simulink model "phi4_m2_vr001_k5_3"  (R2021a)
settings: Solver=FixedStepAuto  StartTime=0.0  StopTime=24.0  FixedStep=1.0  RelTol=1e-3
libraries: deeplib x1
settings Model: Creator=ldy  LastModifiedBy=ldy
settings DataIOCC: SaveFormat=Array  SignalLogging=off  DSMLogging=off
settings DebuggingCC: UnconnectedInputMsg=none  UnconnectedOutputMsg=none  UnconnectedLineMsg=none
settings ModelReferenceCC: EnableRefExpFcnMdlSchedulingChecks=off
settings RTWCC: Description=Generic Real-Time Target  GPUComputeCapability=5.0  DLArmComputeVersion=20.02.1

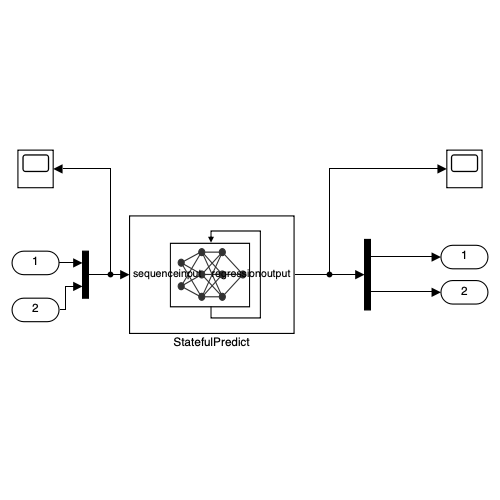
[thumbnail: Simulink's stored preview of the top-level diagram]
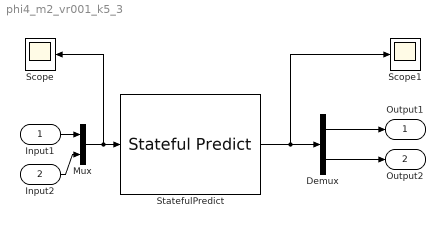
== system phi4_m2_vr001_k5_3 ==
  Input1 : Inport
  Input2 : Inport  Port=2
  Demux : Demux  Outputs=2
  Mux : Mux  Inputs=2
  Scope : Scope
  Scope1 : Scope
  StatefulPredict : deeplib/Stateful Predict  Network=Network from MAT-file  NetworkFunction=untitled  NetworkFilePath=SB4-Synthetic_Benchmark_4/phi4_m2_vr001_k5_3.mat  InputDataFormats={'',''}  SampleTime=1  ForceInterpretedSim=off  EnableDLNetwork=on  LastKnownNetworkFilePath=''  LastKnownNetworkTimeStamp=''
  Output1 : Outport
  Output2 : Outport  Port=2
  wires:
  Input1/1 -> Mux/1
  Input2/1 -> Mux/2
  Mux/1 -> Scope/1, StatefulPredict/1
  Demux/1 -> Output1/1
  Demux/2 -> Output2/1
  StatefulPredict/1 -> Scope1/1, Demux/1
